simulink model "torqueBalancingYoga"  (Simulink 8.8)
settings: Solver=FixedStepDiscrete  StartTime=0.0  StopTime="Config.SIMULATION_TIME "  FixedStep=Config.Ts  RelTol=1e-3  EnableMultiTasking=on
InitFcn:
  | cd(fileparts(which(bdroot)));
  | initTorqueBalancingYoga;
StopFcn:
  | cd(fileparts(which(bdroot)));
  | stopTorqueBalancingYoga;
undefined symbols (not defined in the file or in its folder): bVectorConstraints, Config, ConstraintsMatrix, Gain, Reg, ROBOT_DOF, ROBOT_DOF_FOR_SIMULINK, Sat, Sm
libraries: WBToolboxLibrary x113, simulink x4
(part 2 of 2)

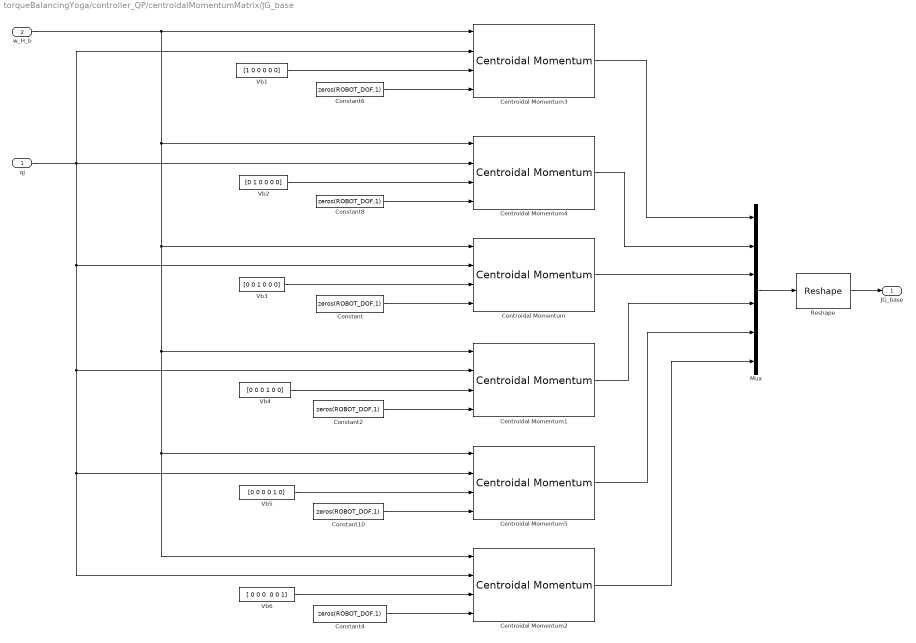
== system torqueBalancingYoga/controller_QP/centroidalMomentumMatrix/JG_base ==
  qj : Inport
  w_H_b : Inport  Port=2
  Centroidal Momentum{,1..5} (6 alike) : WBToolboxLibrary/wholeBodyModel/Dynamics/Centroidal Momentum
  Constant{,2,4,6,8,10} (6 alike) : Constant  Value=zeros(ROBOT_DOF,1)
  Mux : Mux  Inputs=6
  Reshape : Reshape  OutputDimensionality=Customize  OutputDimensions=[6,6]
  Vb1 : Constant  Value=[1 0 0 0 0 0]
  Vb2 : Constant  Value=[0 1 0 0 0 0]
  Vb3 : Constant  Value=[0 0 1 0 0 0]
  Vb4 : Constant  Value=[0 0 0 1 0 0]
  Vb5 : Constant  Value=[0 0 0 0 1 0]
  Vb6 : Constant  Value="[ 0 0 0  0 0 1]"
  JG_base : Outport
  wires:
  Vb1/1 -> Centroidal Momentum3/3
  Vb2/1 -> Centroidal Momentum4/3
  Vb3/1 -> Centroidal Momentum/3
  Vb4/1 -> Centroidal Momentum1/3
  Vb5/1 -> Centroidal Momentum5/3
  Vb6/1 -> Centroidal Momentum2/3
  Constant6/1 -> Centroidal Momentum3/4
  Constant8/1 -> Centroidal Momentum4/4
  Constant/1 -> Centroidal Momentum/4
  Constant2/1 -> Centroidal Momentum1/4
  Constant10/1 -> Centroidal Momentum5/4
  Constant4/1 -> Centroidal Momentum2/4
  qj/1 -> Centroidal Momentum2/2, Centroidal Momentum5/2, Centroidal Momentum1/2, Centroidal Momentum/2, Centroidal Momentum3/2, Centroidal Momentum4/2
  w_H_b/1 -> Centroidal Momentum3/1, Centroidal Momentum2/1, Centroidal Momentum5/1, Centroidal Momentum1/1, Centroidal Momentum/1, Centroidal Momentum4/1
  Centroidal Momentum3/1 -> Mux/1
  Centroidal Momentum4/1 -> Mux/2
  Centroidal Momentum/1 -> Mux/3
  Centroidal Momentum1/1 -> Mux/4
  Centroidal Momentum5/1 -> Mux/5
  Centroidal Momentum2/1 -> Mux/6
  Mux/1 -> Reshape/1
  Reshape/1 -> JG_base/1

== system torqueBalancingYoga/controller_QP/centroidalMomentumMatrix/JG_joints ==
  qj : Inport
  w_H_b : Inport  Port=2
  JG_Larm : Subsystem
  JG_Lleg : Subsystem
  JG_Rarm : Subsystem
  JG_Rleg : Subsystem
  JG_torso : Subsystem
  Matrix Concatenate : Concatenate  NumInputs=5  Mode=Multidimensional array  ConcatenateDimension=2
  JG_joints : Outport
  wires:
  qj/1 -> JG_Rarm/1(qj), JG_Rleg/1(qj), JG_Lleg/1(qj), JG_Larm/1(qj), JG_torso/1(qj)
  w_H_b/1 -> JG_Rarm/2(w _H_b), JG_Rleg/2(w_H_b), JG_Lleg/2(w_H_b), JG_Larm/2(w_H_b), JG_torso/2(w_H_b)
  JG_torso/1(JG_torso) -> Matrix Concatenate/1
  JG_Larm/1(JG_Larm) -> Matrix Concatenate/2
  JG_Rarm/1(JG_Rarm) -> Matrix Concatenate/3
  JG_Lleg/1(JG_Lleg) -> Matrix Concatenate/4
  JG_Rleg/1(JG_Rleg) -> Matrix Concatenate/5
  Matrix Concatenate/1 -> JG_joints/1

== system torqueBalancingYoga/Robot State and References/Internal Coordinator/Base to fixed_link/LFoot to base link transform  ==
  qj : Inport
  inertial : Inport  Port=2
  w_H_link : Inport  Port=3
  w_H_base_fixed : Inport  Port=4
  Fixed base to imu transform : WBToolboxLibrary/wholeBodyModel/Kinematics/Forward Kinematics  frameName=Frames.IMU
  Fixed base to root link transform : WBToolboxLibrary/wholeBodyModel/Kinematics/Forward Kinematics  frameName=Frames.BASE
  Inv\* : Product  Inputs=/*  Multiplication=Matrix(*)
  "Inv\\*  " : Product  Inputs=/*  Multiplication=Matrix(*)
  Neck Position : WBToolboxLibrary/Utilities/Yarp Read  portName=Ports.NECK_POS  signalSize=6  timeout=0.5  blocking=off  timestamp=off  autoconnect=on  errorOnConnection=off
  Switch6 : Switch  Criteria=u2 > Threshold
  USE_IMU4EST_BASE : Constant  Value=Config.USE_IMU4EST_BASE
  fromImuToHomogeousTransformFCN : MATLAB Function  TreatAsAtomicUnit=on
  holder 1 : WBToolboxLibrary/Utilities/holder 
  holder 2 : WBToolboxLibrary/Utilities/holder 
  neck transform : Subsystem
  link_H_b : Outport
  wires:
  Switch6/1 -> link_H_b/1
  "Inv\\*  "/1 -> Switch6/3, fromImuToHomogeousTransformFCN/3(link_H_base)  "link_H_root"
  USE_IMU4EST_BASE/1 -> Switch6/2
  Inv\*/1 -> fromImuToHomogeousTransformFCN/1(imu_H_link), holder 1/1  "imu_H_link"
  holder 2/1 -> fromImuToHomogeousTransformFCN/4(inertial_0)
  Fixed base to imu transform/1 -> Inv\*/1
  holder 1/1 -> fromImuToHomogeousTransformFCN/2(imu_H_link_0)
  qj/1 -> Fixed base to imu transform/2, Fixed base to root link transform/2
  fromImuToHomogeousTransformFCN/1(w_H_b) -> Switch6/1
  Fixed base to root link transform/1 -> "Inv\\*  "/2
  inertial/1 -> holder 2/1, fromImuToHomogeousTransformFCN/5(inertial)
  Neck Position/1 -> neck transform/1(neck port)
  neck transform/1(neck position) -> fromImuToHomogeousTransformFCN/6(neck_pos)
  w_H_link/1 -> "Inv\\*  "/1, Inv\*/2
  w_H_base_fixed/1 -> Fixed base to root link transform/1, Fixed base to imu transform/1

== system torqueBalancingYoga/Robot State and References/Internal Coordinator/Compute State Velocity/Feet Jacobians ==
  qj : Inport
  w_H_b : Inport  Port=2
  Jacobian LFoot : WBToolboxLibrary/wholeBodyModel/Jacobians/Jacobian  frameName=Frames.LEFT_FOOT
  Jacobian RFoot : WBToolboxLibrary/wholeBodyModel/Jacobians/Jacobian  frameName=Frames.RIGHT_FOOT
  J_LFoot : Outport
  J_RFoot : Outport  Port=2
  wires:
  Jacobian LFoot/1 -> J_LFoot/1
  Jacobian RFoot/1 -> J_RFoot/1
  w_H_b/1 -> Jacobian RFoot/1, Jacobian LFoot/1
  qj/1 -> Jacobian LFoot/2, Jacobian RFoot/2

== system torqueBalancingYoga/Robot State and References/State Machine Yoga/Compute State Velocity/Feet Jacobians ==
  qj : Inport
  w_H_b : Inport  Port=2
  Jacobian LFoot : WBToolboxLibrary/wholeBodyModel/Jacobians/Jacobian  frameName=Frames.LEFT_FOOT
  Jacobian RFoot : WBToolboxLibrary/wholeBodyModel/Jacobians/Jacobian  frameName=Frames.RIGHT_FOOT
  J_LFoot : Outport
  J_RFoot : Outport  Port=2
  wires:
  Jacobian LFoot/1 -> J_LFoot/1
  Jacobian RFoot/1 -> J_RFoot/1
  w_H_b/1 -> Jacobian RFoot/1, Jacobian LFoot/1
  qj/1 -> Jacobian LFoot/2, Jacobian RFoot/2

== system torqueBalancingYoga/Robot State and References/State Machine Yoga/Compute base to fixed link transform/LFoot to base link transform  ==
  qj : Inport
  inertial : Inport  Port=2
  w_H_link : Inport  Port=3
  w_H_base_fixed : Inport  Port=4
  Fixed base to imu transform : WBToolboxLibrary/wholeBodyModel/Kinematics/Forward Kinematics  frameName=Frames.IMU
  Fixed base to root link transform : WBToolboxLibrary/wholeBodyModel/Kinematics/Forward Kinematics  frameName=Frames.BASE
  Inv\* : Product  Inputs=/*  Multiplication=Matrix(*)
  "Inv\\*  " : Product  Inputs=/*  Multiplication=Matrix(*)
  Neck Position : WBToolboxLibrary/Utilities/Yarp Read  portName=Ports.NECK_POS  signalSize=6  timeout=0.5  blocking=off  timestamp=off  autoconnect=on  errorOnConnection=off
  Switch6 : Switch  Criteria=u2 > Threshold
  USE_IMU4EST_BASE : Constant  Value=Config.USE_IMU4EST_BASE
  fromImuToHomogeousTransformFCN : MATLAB Function  TreatAsAtomicUnit=on
  holder 1 : WBToolboxLibrary/Utilities/holder 
  holder 2 : WBToolboxLibrary/Utilities/holder 
  neck transform : Subsystem
  link_H_b : Outport
  wires:
  Switch6/1 -> link_H_b/1
  "Inv\\*  "/1 -> Switch6/3, fromImuToHomogeousTransformFCN/3(link_H_base)  "link_H_root"
  USE_IMU4EST_BASE/1 -> Switch6/2
  Inv\*/1 -> fromImuToHomogeousTransformFCN/1(imu_H_link), holder 1/1  "imu_H_link"
  holder 2/1 -> fromImuToHomogeousTransformFCN/4(inertial_0)
  Fixed base to imu transform/1 -> Inv\*/1
  holder 1/1 -> fromImuToHomogeousTransformFCN/2(imu_H_link_0)
  qj/1 -> Fixed base to imu transform/2, Fixed base to root link transform/2
  fromImuToHomogeousTransformFCN/1(w_H_b) -> Switch6/1
  Fixed base to root link transform/1 -> "Inv\\*  "/2
  inertial/1 -> holder 2/1, fromImuToHomogeousTransformFCN/5(inertial)
  Neck Position/1 -> neck transform/1(neck port)
  neck transform/1(neck position) -> fromImuToHomogeousTransformFCN/6(neck_pos)
  w_H_link/1 -> "Inv\\*  "/1, Inv\*/2
  w_H_base_fixed/1 -> Fixed base to root link transform/1, Fixed base to imu transform/1

== system torqueBalancingYoga/Robot State and References/State Machine Yoga/Compute base to fixed link transform/RFoot to base link transform ==
  qj : Inport
  inertial : Inport  Port=2
  w_H_link : Inport  Port=3
  w_H_base_fixed : Inport  Port=4
  Fixed base to imu transform : WBToolboxLibrary/wholeBodyModel/Kinematics/Forward Kinematics  frameName=Frames.IMU
  Fixed base to root link transform : WBToolboxLibrary/wholeBodyModel/Kinematics/Forward Kinematics  frameName=Frames.BASE
  Inv\* : Product  Inputs=/*  Multiplication=Matrix(*)
  "Inv\\*  " : Product  Inputs=/*  Multiplication=Matrix(*)
  Neck Position : WBToolboxLibrary/Utilities/Yarp Read  portName=Ports.NECK_POS  signalSize=6  timeout=0.5  blocking=off  timestamp=off  autoconnect=on  errorOnConnection=off
  Switch6 : Switch  Criteria=u2 > Threshold
  USE_IMU4EST_BASE : Constant  Value=Config.USE_IMU4EST_BASE
  fromImuToHomogeousTransformFCN : MATLAB Function  TreatAsAtomicUnit=on
  holder 1 : WBToolboxLibrary/Utilities/holder 
  holder 2 : WBToolboxLibrary/Utilities/holder 
  neck transform : Subsystem
  link_H_b : Outport
  wires:
  Switch6/1 -> link_H_b/1
  "Inv\\*  "/1 -> Switch6/3, fromImuToHomogeousTransformFCN/3(link_H_base)  "link_H_root"
  USE_IMU4EST_BASE/1 -> Switch6/2
  Inv\*/1 -> fromImuToHomogeousTransformFCN/1(imu_H_link), holder 1/1  "imu_H_link"
  holder 2/1 -> fromImuToHomogeousTransformFCN/4(inertial_0)
  Fixed base to imu transform/1 -> Inv\*/1
  holder 1/1 -> fromImuToHomogeousTransformFCN/2(imu_H_link_0)
  qj/1 -> Fixed base to imu transform/2, Fixed base to root link transform/2
  fromImuToHomogeousTransformFCN/1(w_H_b) -> Switch6/1
  Fixed base to root link transform/1 -> "Inv\\*  "/2
  inertial/1 -> holder 2/1, fromImuToHomogeousTransformFCN/5(inertial)
  Neck Position/1 -> neck transform/1(neck port)
  neck transform/1(neck position) -> fromImuToHomogeousTransformFCN/6(neck_pos)
  w_H_link/1 -> "Inv\\*  "/1, Inv\*/2
  w_H_base_fixed/1 -> Fixed base to root link transform/1, Fixed base to imu transform/1

== system torqueBalancingYoga/controller_QP/Compute angular momentum integral/Compute base to fixed link transform/LFoot to base link transform  ==
  qj : Inport
  inertial : Inport  Port=2
  w_H_link : Inport  Port=3
  w_H_base_fixed : Inport  Port=4
  Fixed base to imu transform : WBToolboxLibrary/wholeBodyModel/Kinematics/Forward Kinematics  frameName=Frames.IMU
  Fixed base to root link transform : WBToolboxLibrary/wholeBodyModel/Kinematics/Forward Kinematics  frameName=Frames.BASE
  Inv\* : Product  Inputs=/*  Multiplication=Matrix(*)
  "Inv\\*  " : Product  Inputs=/*  Multiplication=Matrix(*)
  Neck Position : WBToolboxLibrary/Utilities/Yarp Read  portName=Ports.NECK_POS  signalSize=6  timeout=0.5  blocking=off  timestamp=off  autoconnect=on  errorOnConnection=off
  Switch6 : Switch  Criteria=u2 > Threshold
  USE_IMU4EST_BASE : Constant  Value=Config.USE_IMU4EST_BASE
  fromImuToHomogeousTransformFCN : MATLAB Function  TreatAsAtomicUnit=on
  holder 1 : WBToolboxLibrary/Utilities/holder 
  holder 2 : WBToolboxLibrary/Utilities/holder 
  neck transform : Subsystem
  link_H_b : Outport
  wires:
  Switch6/1 -> link_H_b/1
  "Inv\\*  "/1 -> Switch6/3, fromImuToHomogeousTransformFCN/3(link_H_base)  "link_H_root"
  USE_IMU4EST_BASE/1 -> Switch6/2
  Inv\*/1 -> fromImuToHomogeousTransformFCN/1(imu_H_link), holder 1/1  "imu_H_link"
  holder 2/1 -> fromImuToHomogeousTransformFCN/4(inertial_0)
  Fixed base to imu transform/1 -> Inv\*/1
  holder 1/1 -> fromImuToHomogeousTransformFCN/2(imu_H_link_0)
  qj/1 -> Fixed base to imu transform/2, Fixed base to root link transform/2
  fromImuToHomogeousTransformFCN/1(w_H_b) -> Switch6/1
  Fixed base to root link transform/1 -> "Inv\\*  "/2
  inertial/1 -> holder 2/1, fromImuToHomogeousTransformFCN/5(inertial)
  Neck Position/1 -> neck transform/1(neck port)
  neck transform/1(neck position) -> fromImuToHomogeousTransformFCN/6(neck_pos)
  w_H_link/1 -> "Inv\\*  "/1, Inv\*/2
  w_H_base_fixed/1 -> Fixed base to root link transform/1, Fixed base to imu transform/1

== system torqueBalancingYoga/controller_QP/Compute angular momentum integral/Compute base to fixed link transform/RFoot to base link transform ==
  qj : Inport
  inertial : Inport  Port=2
  w_H_link : Inport  Port=3
  w_H_base_fixed : Inport  Port=4
  Fixed base to imu transform : WBToolboxLibrary/wholeBodyModel/Kinematics/Forward Kinematics  frameName=Frames.IMU
  Fixed base to root link transform : WBToolboxLibrary/wholeBodyModel/Kinematics/Forward Kinematics  frameName=Frames.BASE
  Inv\* : Product  Inputs=/*  Multiplication=Matrix(*)
  "Inv\\*  " : Product  Inputs=/*  Multiplication=Matrix(*)
  Neck Position : WBToolboxLibrary/Utilities/Yarp Read  portName=Ports.NECK_POS  signalSize=6  timeout=0.5  blocking=off  timestamp=off  autoconnect=on  errorOnConnection=off
  Switch6 : Switch  Criteria=u2 > Threshold
  USE_IMU4EST_BASE : Constant  Value=Config.USE_IMU4EST_BASE
  fromImuToHomogeousTransformFCN : MATLAB Function  TreatAsAtomicUnit=on
  holder 1 : WBToolboxLibrary/Utilities/holder 
  holder 2 : WBToolboxLibrary/Utilities/holder 
  neck transform : Subsystem
  link_H_b : Outport
  wires:
  Switch6/1 -> link_H_b/1
  "Inv\\*  "/1 -> Switch6/3, fromImuToHomogeousTransformFCN/3(link_H_base)  "link_H_root"
  USE_IMU4EST_BASE/1 -> Switch6/2
  Inv\*/1 -> fromImuToHomogeousTransformFCN/1(imu_H_link), holder 1/1  "imu_H_link"
  holder 2/1 -> fromImuToHomogeousTransformFCN/4(inertial_0)
  Fixed base to imu transform/1 -> Inv\*/1
  holder 1/1 -> fromImuToHomogeousTransformFCN/2(imu_H_link_0)
  qj/1 -> Fixed base to imu transform/2, Fixed base to root link transform/2
  fromImuToHomogeousTransformFCN/1(w_H_b) -> Switch6/1
  Fixed base to root link transform/1 -> "Inv\\*  "/2
  inertial/1 -> holder 2/1, fromImuToHomogeousTransformFCN/5(inertial)
  Neck Position/1 -> neck transform/1(neck port)
  neck transform/1(neck position) -> fromImuToHomogeousTransformFCN/6(neck_pos)
  w_H_link/1 -> "Inv\\*  "/1, Inv\*/2
  w_H_base_fixed/1 -> Fixed base to root link transform/1, Fixed base to imu transform/1

== system torqueBalancingYoga/controller_QP/Compute joint torques/QPSolver/Visualize eventual QP failures ==
  exitFlagQP : Inport
  state : Inport  Port=2
  Enable : EnablePort
  "QP status (0: no failure, 1: not using)" : Scope  NumInputPorts=2
  wires:
  exitFlagQP/1 -> "QP status (0: no failure, 1: not using)"/1  "exitFlagQP"
  state/1 -> "QP status (0: no failure, 1: not using)"/2

== system torqueBalancingYoga/controller_QP/centroidalMomentumMatrix/JG_joints/JG_Larm ==
  qj : Inport
  w_H_b : Inport  Port=2
  Centroidal Momentum{,1,3..4} (4 alike) : WBToolboxLibrary/wholeBodyModel/Dynamics/Centroidal Momentum
  Constant : Constant  Value=eye(ROBOT_DOF)
  Constant{1..3,6} (4 alike) : Constant  Value=zeros(6,1)
  Mux : Mux
  Reshape : Reshape  OutputDimensionality=Customize  OutputDimensions=[6,4]
  Selector : Selector  NumberOfDimensions=2  InputPortWidth=3  IndexOptions=Index vector (dialog),Select all  Indices=[4],1  OutputSizes=1,1
  Selector1 : Selector  NumberOfDimensions=2  InputPortWidth=3  IndexOptions=Index vector (dialog),Select all  Indices=[5],1  OutputSizes=1,1
  Selector2 : Selector  NumberOfDimensions=2  InputPortWidth=3  IndexOptions=Index vector (dialog),Select all  Indices=[6],1  OutputSizes=1,1
  Selector3 : Selector  NumberOfDimensions=2  InputPortWidth=3  IndexOptions=Index vector (dialog),Select all  Indices=[7],1  OutputSizes=1,1
  JG_Larm : Outport
  wires:
  Constant6/1 -> Centroidal Momentum3/3
  Constant1/1 -> Centroidal Momentum4/3
  Constant3/1 -> Centroidal Momentum/3
  Constant2/1 -> Centroidal Momentum1/3
  qj/1 -> Centroidal Momentum4/2, Centroidal Momentum3/2, Centroidal Momentum1/2, Centroidal Momentum/2
  w_H_b/1 -> Centroidal Momentum1/1, Centroidal Momentum/1, Centroidal Momentum3/1, Centroidal Momentum4/1
  Constant/1 -> Selector3/1, Selector2/1, Selector1/1, Selector/1
  Selector/1 -> Centroidal Momentum3/4
  Selector1/1 -> Centroidal Momentum4/4
  Selector2/1 -> Centroidal Momentum/4
  Selector3/1 -> Centroidal Momentum1/4
  Centroidal Momentum/1 -> Mux/3
  Centroidal Momentum3/1 -> Mux/1
  Centroidal Momentum4/1 -> Mux/2
  Centroidal Momentum1/1 -> Mux/4
  Mux/1 -> Reshape/1
  Reshape/1 -> JG_Larm/1

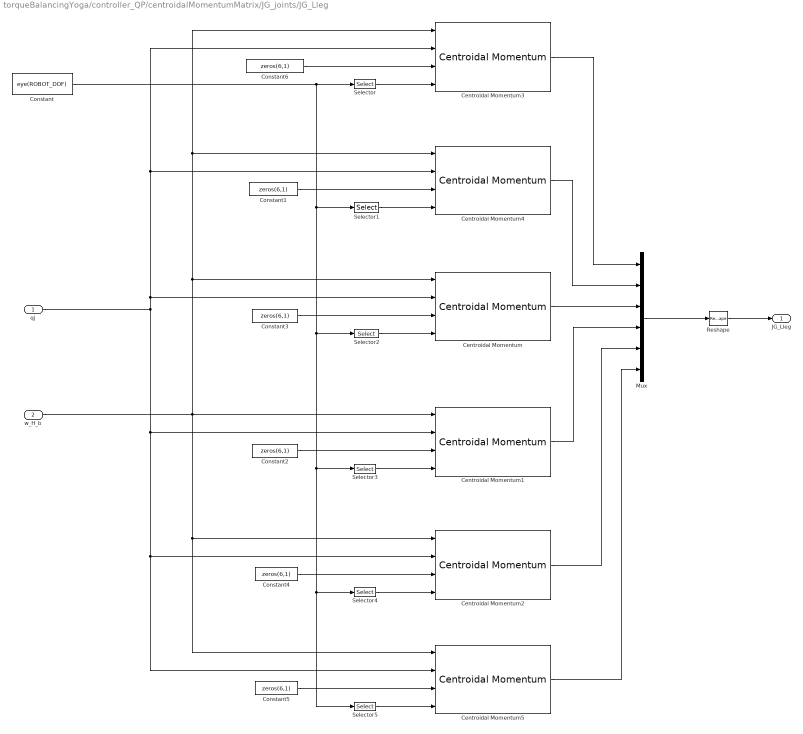
== system torqueBalancingYoga/controller_QP/centroidalMomentumMatrix/JG_joints/JG_Lleg ==
  qj : Inport
  w_H_b : Inport  Port=2
  Centroidal Momentum{,1..5} (6 alike) : WBToolboxLibrary/wholeBodyModel/Dynamics/Centroidal Momentum
  Constant : Constant  Value=eye(ROBOT_DOF)
  Constant{1..6} (6 alike) : Constant  Value=zeros(6,1)
  Mux : Mux  Inputs=6
  Reshape : Reshape  OutputDimensionality=Customize  OutputDimensions=[6,6]
  Selector : Selector  NumberOfDimensions=2  InputPortWidth=3  IndexOptions=Index vector (dialog),Select all  Indices=[12],1  OutputSizes=1,1
  Selector1 : Selector  NumberOfDimensions=2  InputPortWidth=3  IndexOptions=Index vector (dialog),Select all  Indices=[13],1  OutputSizes=1,1
  Selector2 : Selector  NumberOfDimensions=2  InputPortWidth=3  IndexOptions=Index vector (dialog),Select all  Indices=[14],1  OutputSizes=1,1
  Selector3 : Selector  NumberOfDimensions=2  InputPortWidth=3  IndexOptions=Index vector (dialog),Select all  Indices=[15],1  OutputSizes=1,1
  Selector4 : Selector  NumberOfDimensions=2  InputPortWidth=3  IndexOptions=Index vector (dialog),Select all  Indices=[16],1  OutputSizes=1,1
  Selector5 : Selector  NumberOfDimensions=2  InputPortWidth=3  IndexOptions=Index vector (dialog),Select all  Indices=[17],1  OutputSizes=1,1
  JG_Lleg : Outport
  wires:
  Constant6/1 -> Centroidal Momentum3/3
  Constant1/1 -> Centroidal Momentum4/3
  Constant3/1 -> Centroidal Momentum/3
  Constant4/1 -> Centroidal Momentum2/3
  Constant2/1 -> Centroidal Momentum1/3
  qj/1 -> Centroidal Momentum4/2, Centroidal Momentum3/2, Centroidal Momentum/2, Centroidal Momentum5/2, Centroidal Momentum2/2, Centroidal Momentum1/2
  Constant/1 -> Selector5/1, Selector4/1, Selector3/1, Selector2/1, Selector1/1, Selector/1
  Selector/1 -> Centroidal Momentum3/4
  Selector1/1 -> Centroidal Momentum4/4
  Selector2/1 -> Centroidal Momentum/4
  Selector3/1 -> Centroidal Momentum1/4
  Selector4/1 -> Centroidal Momentum2/4
  Centroidal Momentum/1 -> Mux/3
  Centroidal Momentum3/1 -> Mux/1
  Centroidal Momentum4/1 -> Mux/2
  Centroidal Momentum1/1 -> Mux/4
  Centroidal Momentum2/1 -> Mux/5
  Mux/1 -> Reshape/1
  Reshape/1 -> JG_Lleg/1
  Constant5/1 -> Centroidal Momentum5/3
  Selector5/1 -> Centroidal Momentum5/4
  Centroidal Momentum5/1 -> Mux/6
  w_H_b/1 -> Centroidal Momentum1/1, Centroidal Momentum5/1, Centroidal Momentum2/1, Centroidal Momentum/1, Centroidal Momentum3/1, Centroidal Momentum4/1

== system torqueBalancingYoga/controller_QP/centroidalMomentumMatrix/JG_joints/JG_Rarm ==
  qj : Inport
  w _H_b : Inport  Port=2
  Centroidal Momentum{,1,3..4} (4 alike) : WBToolboxLibrary/wholeBodyModel/Dynamics/Centroidal Momentum
  Constant : Constant  Value=eye(ROBOT_DOF)
  Constant{1..3,6} (4 alike) : Constant  Value=zeros(6,1)
  Mux : Mux
  Reshape : Reshape  OutputDimensionality=Customize  OutputDimensions=[6,4]
  Selector : Selector  NumberOfDimensions=2  InputPortWidth=3  IndexOptions=Index vector (dialog),Select all  Indices=[8],1  OutputSizes=1,1
  Selector1 : Selector  NumberOfDimensions=2  InputPortWidth=3  IndexOptions=Index vector (dialog),Select all  Indices=[9],1  OutputSizes=1,1
  Selector2 : Selector  NumberOfDimensions=2  InputPortWidth=3  IndexOptions=Index vector (dialog),Select all  Indices=[10],1  OutputSizes=1,1
  Selector3 : Selector  NumberOfDimensions=2  InputPortWidth=3  IndexOptions=Index vector (dialog),Select all  Indices=[11],1  OutputSizes=1,1
  JG_Rarm : Outport
  wires:
  Constant6/1 -> Centroidal Momentum3/3
  Constant1/1 -> Centroidal Momentum4/3
  Constant3/1 -> Centroidal Momentum/3
  Constant2/1 -> Centroidal Momentum1/3
  qj/1 -> Centroidal Momentum4/2, Centroidal Momentum3/2, Centroidal Momentum1/2, Centroidal Momentum/2
  w _H_b/1 -> Centroidal Momentum1/1, Centroidal Momentum/1, Centroidal Momentum3/1, Centroidal Momentum4/1
  Constant/1 -> Selector3/1, Selector2/1, Selector1/1, Selector/1
  Selector/1 -> Centroidal Momentum3/4
  Selector1/1 -> Centroidal Momentum4/4
  Selector2/1 -> Centroidal Momentum/4
  Selector3/1 -> Centroidal Momentum1/4
  Centroidal Momentum/1 -> Mux/3
  Centroidal Momentum3/1 -> Mux/1
  Centroidal Momentum4/1 -> Mux/2
  Centroidal Momentum1/1 -> Mux/4
  Mux/1 -> Reshape/1
  Reshape/1 -> JG_Rarm/1

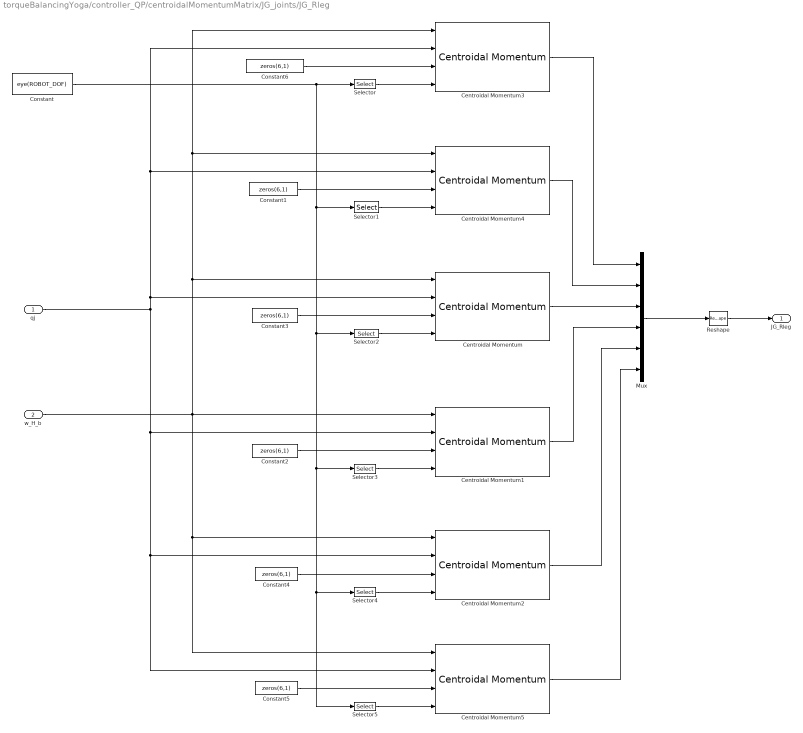
== system torqueBalancingYoga/controller_QP/centroidalMomentumMatrix/JG_joints/JG_Rleg ==
  qj : Inport
  w_H_b : Inport  Port=2
  Centroidal Momentum{,1..5} (6 alike) : WBToolboxLibrary/wholeBodyModel/Dynamics/Centroidal Momentum
  Constant : Constant  Value=eye(ROBOT_DOF)
  Constant{1..6} (6 alike) : Constant  Value=zeros(6,1)
  Mux : Mux  Inputs=6
  Reshape : Reshape  OutputDimensionality=Customize  OutputDimensions=[6,6]
  Selector : Selector  NumberOfDimensions=2  InputPortWidth=3  IndexOptions=Index vector (dialog),Select all  Indices=[18],1  OutputSizes=1,1
  Selector1 : Selector  NumberOfDimensions=2  InputPortWidth=3  IndexOptions=Index vector (dialog),Select all  Indices=[19],1  OutputSizes=1,1
  Selector2 : Selector  NumberOfDimensions=2  InputPortWidth=3  IndexOptions=Index vector (dialog),Select all  Indices=[20],1  OutputSizes=1,1
  Selector3 : Selector  NumberOfDimensions=2  InputPortWidth=3  IndexOptions=Index vector (dialog),Select all  Indices=[21],1  OutputSizes=1,1
  Selector4 : Selector  NumberOfDimensions=2  InputPortWidth=3  IndexOptions=Index vector (dialog),Select all  Indices=[22],1  OutputSizes=1,1
  Selector5 : Selector  NumberOfDimensions=2  InputPortWidth=3  IndexOptions=Index vector (dialog),Select all  Indices=[23],1  OutputSizes=1,1
  JG_Rleg : Outport
  wires:
  Constant6/1 -> Centroidal Momentum3/3
  Constant1/1 -> Centroidal Momentum4/3
  Constant3/1 -> Centroidal Momentum/3
  Constant4/1 -> Centroidal Momentum2/3
  Constant2/1 -> Centroidal Momentum1/3
  qj/1 -> Centroidal Momentum4/2, Centroidal Momentum3/2, Centroidal Momentum/2, Centroidal Momentum5/2, Centroidal Momentum2/2, Centroidal Momentum1/2
  w_H_b/1 -> Centroidal Momentum1/1, Centroidal Momentum5/1, Centroidal Momentum2/1, Centroidal Momentum/1, Centroidal Momentum3/1, Centroidal Momentum4/1
  Constant/1 -> Selector5/1, Selector4/1, Selector3/1, Selector2/1, Selector1/1, Selector/1
  Selector/1 -> Centroidal Momentum3/4
  Selector1/1 -> Centroidal Momentum4/4
  Selector2/1 -> Centroidal Momentum/4
  Selector3/1 -> Centroidal Momentum1/4
  Selector4/1 -> Centroidal Momentum2/4
  Centroidal Momentum/1 -> Mux/3
  Centroidal Momentum3/1 -> Mux/1
  Centroidal Momentum4/1 -> Mux/2
  Centroidal Momentum1/1 -> Mux/4
  Centroidal Momentum2/1 -> Mux/5
  Mux/1 -> Reshape/1
  Reshape/1 -> JG_Rleg/1
  Constant5/1 -> Centroidal Momentum5/3
  Selector5/1 -> Centroidal Momentum5/4
  Centroidal Momentum5/1 -> Mux/6

== system torqueBalancingYoga/controller_QP/centroidalMomentumMatrix/JG_joints/JG_torso ==
  qj : Inport
  w_H_b : Inport  Port=2
  Centroidal Momentum : WBToolboxLibrary/wholeBodyModel/Dynamics/Centroidal Momentum
  Centroidal Momentum3 : WBToolboxLibrary/wholeBodyModel/Dynamics/Centroidal Momentum
  Centroidal Momentum4 : WBToolboxLibrary/wholeBodyModel/Dynamics/Centroidal Momentum
  Constant : Constant  Value=eye(ROBOT_DOF)
  Constant1 : Constant  Value=zeros(6,1)
  Constant3 : Constant  Value=zeros(6,1)
  Constant6 : Constant  Value=zeros(6,1)
  Mux : Mux  Inputs=3
  Reshape : Reshape  OutputDimensionality=Customize  OutputDimensions=[6,3]
  Selector : Selector  NumberOfDimensions=2  InputPortWidth=3  IndexOptions=Index vector (dialog),Select all  Indices=[1],1  OutputSizes=1,1
  Selector1 : Selector  NumberOfDimensions=2  InputPortWidth=3  IndexOptions=Index vector (dialog),Select all  Indices=[2],1  OutputSizes=1,1
  Selector2 : Selector  NumberOfDimensions=2  InputPortWidth=3  IndexOptions=Index vector (dialog),Select all  Indices=[3],1  OutputSizes=1,1
  JG_torso : Outport
  wires:
  qj/1 -> Centroidal Momentum3/2, Centroidal Momentum4/2, Centroidal Momentum/2
  w_H_b/1 -> Centroidal Momentum/1, Centroidal Momentum4/1, Centroidal Momentum3/1
  Centroidal Momentum3/1 -> Mux/1
  Centroidal Momentum4/1 -> Mux/2
  Centroidal Momentum/1 -> Mux/3
  Constant6/1 -> Centroidal Momentum3/3
  Constant1/1 -> Centroidal Momentum4/3
  Constant3/1 -> Centroidal Momentum/3
  Mux/1 -> Reshape/1
  Constant/1 -> Selector2/1, Selector1/1, Selector/1
  Selector/1 -> Centroidal Momentum3/4
  Selector1/1 -> Centroidal Momentum4/4
  Selector2/1 -> Centroidal Momentum/4
  Reshape/1 -> JG_torso/1

== system torqueBalancingYoga/Robot State and References/Internal Coordinator/Base to fixed_link/LFoot to base link transform /neck transform ==
  neck port : Inport
  Constant : Constant  Value=zeros(3,1)
  Gain : Gain  Gain=pi/180
  Selector1 : Selector  InputPortWidth=6  IndexOptions=Index vector (dialog)  Indices=[1:3]  OutputSizes=1
  Switch : Switch  Criteria=u2 > Threshold
  USE_IMU4EST_BASE1 : Constant  Value=Config.CORRECT_NECK_IMU
  neck position : Outport
  wires:
  neck port/1 -> Gain/1
  USE_IMU4EST_BASE1/1 -> Switch/2
  Switch/1 -> neck position/1
  Gain/1 -> Selector1/1
  Constant/1 -> Switch/3
  Selector1/1 -> Switch/1  "neck pos"

== system torqueBalancingYoga/Robot State and References/State Machine Yoga/Compute base to fixed link transform/LFoot to base link transform /neck transform ==
  neck port : Inport
  Constant : Constant  Value=zeros(3,1)
  Gain : Gain  Gain=pi/180
  Selector1 : Selector  InputPortWidth=6  IndexOptions=Index vector (dialog)  Indices=[1:3]  OutputSizes=1
  Switch : Switch  Criteria=u2 > Threshold
  USE_IMU4EST_BASE1 : Constant  Value=Config.CORRECT_NECK_IMU
  neck position : Outport
  wires:
  neck port/1 -> Gain/1
  USE_IMU4EST_BASE1/1 -> Switch/2
  Switch/1 -> neck position/1
  Gain/1 -> Selector1/1
  Constant/1 -> Switch/3
  Selector1/1 -> Switch/1  "neck pos"

== system torqueBalancingYoga/Robot State and References/State Machine Yoga/Compute base to fixed link transform/RFoot to base link transform/neck transform ==
  neck port : Inport
  Constant : Constant  Value=zeros(3,1)
  Gain : Gain  Gain=pi/180
  Selector1 : Selector  InputPortWidth=6  IndexOptions=Index vector (dialog)  Indices=[1:3]  OutputSizes=1
  Switch : Switch  Criteria=u2 > Threshold
  USE_IMU4EST_BASE1 : Constant  Value=Config.CORRECT_NECK_IMU
  neck position : Outport
  wires:
  neck port/1 -> Gain/1
  USE_IMU4EST_BASE1/1 -> Switch/2
  Switch/1 -> neck position/1
  Gain/1 -> Selector1/1
  Constant/1 -> Switch/3
  Selector1/1 -> Switch/1  "neck pos"

== system torqueBalancingYoga/controller_QP/Compute angular momentum integral/Compute base to fixed link transform/LFoot to base link transform /neck transform ==
  neck port : Inport
  Constant : Constant  Value=zeros(3,1)
  Gain : Gain  Gain=pi/180
  Selector1 : Selector  InputPortWidth=6  IndexOptions=Index vector (dialog)  Indices=[1:3]  OutputSizes=1
  Switch : Switch  Criteria=u2 > Threshold
  USE_IMU4EST_BASE1 : Constant  Value=Config.CORRECT_NECK_IMU
  neck position : Outport
  wires:
  neck port/1 -> Gain/1
  USE_IMU4EST_BASE1/1 -> Switch/2
  Switch/1 -> neck position/1
  Gain/1 -> Selector1/1
  Constant/1 -> Switch/3
  Selector1/1 -> Switch/1  "neck pos"

== system torqueBalancingYoga/controller_QP/Compute angular momentum integral/Compute base to fixed link transform/RFoot to base link transform/neck transform ==
  neck port : Inport
  Constant : Constant  Value=zeros(3,1)
  Gain : Gain  Gain=pi/180
  Selector1 : Selector  InputPortWidth=6  IndexOptions=Index vector (dialog)  Indices=[1:3]  OutputSizes=1
  Switch : Switch  Criteria=u2 > Threshold
  USE_IMU4EST_BASE1 : Constant  Value=Config.CORRECT_NECK_IMU
  neck position : Outport
  wires:
  neck port/1 -> Gain/1
  USE_IMU4EST_BASE1/1 -> Switch/2
  Switch/1 -> neck position/1
  Gain/1 -> Selector1/1
  Constant/1 -> Switch/3
  Selector1/1 -> Switch/1  "neck pos"

== matlab function controller_QP/Compute angular momentum integral/Compute base to fixed link transform/LFoot to base link transform /fromImuToHomogeousTransformFCN ==
  data: imu_H_link input double; imu_H_link_0 input double; link_H_base input double; inertial_0 input double; inertial input double; neck_pos input double; w_H_b output double; Config parameter double
function w_H_b = worldToBaseTransformWithIMUFCN(imu_H_link,imu_H_link_0,link_H_base,inertial_0,inertial,neck_pos,Config)

    w_H_b = worldToBaseTransformWithIMU(imu_H_link,imu_H_link_0,link_H_base,inertial_0,inertial,neck_pos,Config);

end

== matlab function Robot State and References/Internal Coordinator/Base to fixed_link/LFoot to base link transform /fromImuToHomogeousTransformFCN ==
  data: imu_H_link input double; imu_H_link_0 input double; link_H_base input double; inertial_0 input double; inertial input double; neck_pos input double; w_H_b output double; Config parameter double
function w_H_b = worldToBaseTransformWithIMUFCN(imu_H_link,imu_H_link_0,link_H_base,inertial_0,inertial,neck_pos,Config)

    w_H_b = worldToBaseTransformWithIMU(imu_H_link,imu_H_link_0,link_H_base,inertial_0,inertial,neck_pos,Config);

end

== matlab function Robot State and References/State Machine Yoga/Compute base to fixed link transform/RFoot to base link transform/fromImuToHomogeousTransformFCN ==
  data: imu_H_link input double; imu_H_link_0 input double; link_H_base input double; inertial_0 input double; inertial input double; neck_pos input double; w_H_b output double; Config parameter double
function w_H_b = worldToBaseTransformWithIMUFCN(imu_H_link,imu_H_link_0,link_H_base,inertial_0,inertial,neck_pos,Config)

    w_H_b = worldToBaseTransformWithIMU(imu_H_link,imu_H_link_0,link_H_base,inertial_0,inertial,neck_pos,Config);

end

== matlab function controller_QP/Compute angular momentum integral/Compute base to fixed link transform/RFoot to base link transform/fromImuToHomogeousTransformFCN ==
  data: imu_H_link input double; imu_H_link_0 input double; link_H_base input double; inertial_0 input double; inertial input double; neck_pos input double; w_H_b output double; Config parameter double
function w_H_b = worldToBaseTransformWithIMUFCN(imu_H_link,imu_H_link_0,link_H_base,inertial_0,inertial,neck_pos,Config)

    w_H_b = worldToBaseTransformWithIMU(imu_H_link,imu_H_link_0,link_H_base,inertial_0,inertial,neck_pos,Config);

end

== matlab function Robot State and References/Internal Coordinator/Compute State Velocity/Compute Base Velocity ==
  data: J_LeftFoot input double; J_RightFoot input double; feetInContact input double; nu_b output double; qjDot input double; Reg parameter double
function nu_b = computeBaseVelocityFCN(J_LeftFoot, J_RightFoot, feetInContact, qjDot, Reg)

    nu_b = computeBaseVelocity(J_LeftFoot, J_RightFoot, feetInContact, qjDot, Reg);
end

== matlab function Dynamics and Kinematics/Dynamics/Add motors reflected inertias/Add motor reflected inertias ==
  data: M input double; M_with_inertia output double; Config parameter double
function M_with_inertia = addMotorsInertiaFCN(M,Config)

    M_with_inertia = addMotorsInertia(M,Config);

end

== matlab function Robot State and References/State Machine Yoga/Compute State Velocity/Compute Base Velocity ==
  data: J_LeftFoot input double; J_RightFoot input double; feetInContact input double; nu_b output double; qjDot input double; Reg parameter double
function nu_b = computeBaseVelocityFCN(J_LeftFoot, J_RightFoot, feetInContact, qjDot, Reg)

    nu_b = computeBaseVelocity(J_LeftFoot, J_RightFoot, feetInContact, qjDot, Reg);
end

== matlab function Robot State and References/State Machine Yoga/Compute base to fixed link transform/LFoot to base link transform /fromImuToHomogeousTransformFCN ==
  data: imu_H_link input double; imu_H_link_0 input double; link_H_base input double; inertial_0 input double; inertial input double; neck_pos input double; w_H_b output double; Config parameter double
function w_H_b = worldToBaseTransformWithIMUFCN(imu_H_link,imu_H_link_0,link_H_base,inertial_0,inertial,neck_pos,Config)

    w_H_b = worldToBaseTransformWithIMU(imu_H_link,imu_H_link_0,link_H_base,inertial_0,inertial,neck_pos,Config);

end

== matlab function controller_QP/Compute joint torques (motor reflected inertia)/(transpose(T*Gamma))^{-1}*I_m*(T*Gamma)^{-1} ==
  data: reflectedInertia output double; Config parameter double
function reflectedInertia  = computeMotorsInertiaFCN(Config)

    [reflectedInertia] = computeMotorsInertia(Config);

end

== matlab function Robot State and References/Internal Coordinator/Reference Generator CoM ==
  data: pos_CoM_0 input double; t input double; references_CoM output double; Config parameter double
function references_CoM = referenceGeneratorCoMFCN(pos_CoM_0, t, Config)

    references_CoM = referenceGeneratorCoM(pos_CoM_0, t, Config);
end

== matlab function Robot State and References/State Machine Yoga/stateMachineYogaFCN ==
  data: wrench_rightFoot input double; wrench_leftFoot input double; w_H_b output double; CoM_des output double; qj_des output double; constraints output double; CoM_0 input double; q0 input double; l_sole_CoM input double; r_sole_CoM input double; qj input double; t input double; l_sole_H_b input double; r_sole_H_b input double; Sm parameter double; impedances output double; KPCoM output double; KDCoM output double; Gain parameter double; currentState output double; jointsSmoothingTime output double
function [w_H_b, CoM_des, qj_des, constraints, impedances, KPCoM, KDCoM, currentState, jointsSmoothingTime] = ...
          stateMachineYogaFCN(wrench_rightFoot, wrench_leftFoot, CoM_0, q0, l_sole_CoM, r_sole_CoM, qj, t, l_sole_H_b, r_sole_H_b, Sm, Gain)
 
    [w_H_b, CoM_des, qj_des, constraints, impedances, KPCoM, KDCoM, currentState, jointsSmoothingTime] = ...
        stateMachineYoga(CoM_0, q0, l_sole_CoM, r_sole_CoM, qj, t, wrench_rightFoot, wrench_leftFoot, l_sole_H_b, r_sole_H_b, Sm, Gain); 
end

== matlab function controller_QP/Balancing Controller  ==
  data: tauModel output double; Sigma output double; NA output double; fHdotDesC1C2 output double; HessianMatrixQP1Foot output double; gradientQP1Foot output double; ConstraintsMatrixQP1Foot output double; bVectorConstraintsQp1Foot output double; HessianMatrixQP2Feet output double; gradientQP2Feet output double; ConstraintsMatrixQP2Feet output double; bVectorConstraintsQp2Feet output double; constraints input double; ROBOT_DOF_FOR_SIMULINK input double; ConstraintsMatrix input double; bVectorConstraints input double; qj input double; qjDes input double; nu input double; M input double; h input double; H input double; intHw input double; w_H_l_sole input double; w_H_r_sole input double; JL input double; JR input double; dJLv input double; dJRv input double; xCoM input double; J_CoM input double; desired_x_dx_ddx_CoM input double; gainsPCOM input double; gainsDCOM input double; impedances input double; qjDesDot input double; JG input double; errorCoM output double; f_noQP output double; Gain parameter double; Reg parameter double; HError output double; HDotDes output double; HDotDes_test output double; alpha output double; JcMinvJct output double
function [tauModel, Sigma, NA, fHdotDesC1C2, ...
          HessianMatrixQP1Foot, gradientQP1Foot, ConstraintsMatrixQP1Foot, bVectorConstraintsQp1Foot, ...
          HessianMatrixQP2Feet, gradientQP2Feet, ConstraintsMatrixQP2Feet, bVectorConstraintsQp2Feet, ...
          errorCoM, f_noQP, HError, HDotDes, HDotDes_test,alpha,JcMinvJct] = ...
              balancingControllerYogaFCN(constraints, ROBOT_DOF_FOR_SIMULINK, ConstraintsMatrix, bVectorConstraints, ...
                  qj, qjDes, nu, M, h, H, intHw, w_H_l_sole, w_H_r_sole, JL, JR, dJLv, dJRv, xCoM, J_CoM, desired_x_dx_ddx_CoM, ...
                  gainsPCOM, gainsDCOM, impedances, qjDesDot, JG, Gain, Reg)
          
    [tauModel, Sigma, NA, fHdotDesC1C2, ...
          HessianMatrixQP1Foot, gradientQP1Foot, ConstraintsMatrixQP1Foot, bVectorConstraintsQp1Foot, ...
          HessianMatrixQP2Feet, gradientQP2Feet, ConstraintsMatrixQP2Feet, bVectorConstraintsQp2Feet, ...
          errorCoM, f_noQP, HError, HDotDes, HDotDes_test,alpha,JcMinvJct] = ...
              balancingControllerYogaFriction(constraints, ROBOT_DOF_FOR_SIMULINK, ConstraintsMatrix, bVectorConstraints, ...
                  qj, qjDes, nu, M, h, H, intHw, w_H_l_sole, w_H_r_sole, JL, JR, dJLv, dJRv, xCoM, J_CoM, desired_x_dx_ddx_CoM, ...
                  gainsPCOM, gainsDCOM, impedances, qjDesDot, JG, Gain, Reg);
end

== matlab function emergency stop: joint limits/MATLAB Function ==
  data: umin input double; umax input double; u input double; inRange output double; tol input double
function inRange = checkRangeFCN(umin, umax, u, tol)

     inRange = checkRange(umin, umax, u, tol);
end

== matlab function controller_QP/Compute angular momentum integral/choose base to world transform ==
  data: state input double; booleanState output double
function booleanState = footOnGround(state)

    % output: a boolean variable whose value is 1 if the foot on ground is left
    % foot, and 0 if the foot on ground is the right foot. If both feet are on
    % ground, the variable is setted to 1.

    % states in which right foot is on ground: 9,10,11,12
    booleanState = 1;

    if state == 9 || state == 10 || state == 11 || state == 12

        booleanState = 0;
    end
end

== matlab function controller_QP/Compute angular momentum integral/References for H ==
  data: qjErr input double; JL input double; JR input double; nu_b_equivalent output double; Reg parameter double; activeFeetConstraints input double
function nu_b_equivalent = generateReferencesForH_FCN(qjErr, JL, JR, Reg, activeFeetConstraints)

    if activeFeetConstraints(1) == 1
    
        pinvJb          = (JL(:,1:6)'*JL(:,1:6) + Reg.pinvDamp_nu_b*eye(6))\JL(:,1:6)';
        nu_b_equivalent = -pinvJb*JL(:,7:end)*qjErr;
    else
    
        pinvJb          = (JR(:,1:6)'*JR(:,1:6) + Reg.pinvDamp_nu_b*eye(6))\JR(:,1:6)';
        nu_b_equivalent = -pinvJb*JR(:,7:end)*qjErr;
    end
end
